simulink model "raspberry_pi_interface"  (R2023a)
settings: Solver=FixedStepDiscrete  StartTime=0.0  StopTime=inf  FixedStep=0.005  RelTol=1e-3  EnableMultiTasking=on
libraries: raspberrypiNetworklib x2, etargetslib x1
settings Model: SimulationMode=external  ExtModeTrigDuration=2  Creator=somml  LastModifiedBy=somml
settings SolverCC: AlgebraicLoopSolver=TrustRegion  PositivePriorityOrder=on
settings DataIOCC: ReturnWorkspaceOutputs=off
settings OptimizationCC: MaxStackSize=64
settings DebuggingCC: ParameterTunabilityLossMsg=error  UnconnectedInputMsg=warning  UnconnectedOutputMsg=warning  UnconnectedLineMsg=warning  ArithmeticOperatorsInVariantConditions=warning
settings HardwareCC: ProdBitPerPointer=32  ProdBitPerSizeT=32  ProdBitPerPtrDiffT=32  ProdLargestAtomicInteger=Long  ProdLargestAtomicFloat=Double  ProdWordSize=32  ProdHWDeviceType=ARM Compatible->ARM Cortex  UseEmbeddedCoderFeatures=off
settings ModelReferenceCC: EnableRefExpFcnMdlSchedulingChecks=on
settings SFSimCC: SimUseLocalCustomCode=off  CustomCodeUndefinedFunction=UseInterfaceOnly
settings RTWCC: Description=Embedded Coder  SystemTargetFile=ert.tlc  HardwareBoard=Raspberry Pi  TLCOptions="-aInlineSetEventsForThisBaseRateFcn=TLC_FALSE -aSuppressMultiTaskScheduler=TLC_FALSE  -aRateBasedStepFcn=0"  TemplateMakefile=ert_default_tmf  GenerateReport=on  RTWUseLocalCustomCode=off  Toolchain=GNU GCC Embedded Linux  BuildConfiguration=Faster Runs  LaunchReport=on  DLArmComputeVersion=19.05
settings CodeAppCC: ForceParamTrailComments=on  OperatorAnnotations=on  StateflowObjectComments=on  MATLABSourceComments=on
settings ERTTargetCC: TargetLangStandard=C99 (ISO)  ERTCustomFileBanners=off  SupportContinuousTime=on  SupportNonInlinedSFcns=on  RemoveResetFunc=off  SupportVariableSizeSignals=on  ModelStepFunctionPrototypeControlCompliant=off

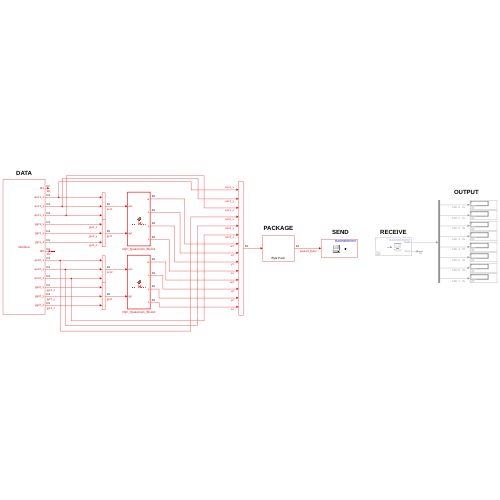
[thumbnail: Simulink's stored preview of the top-level diagram]
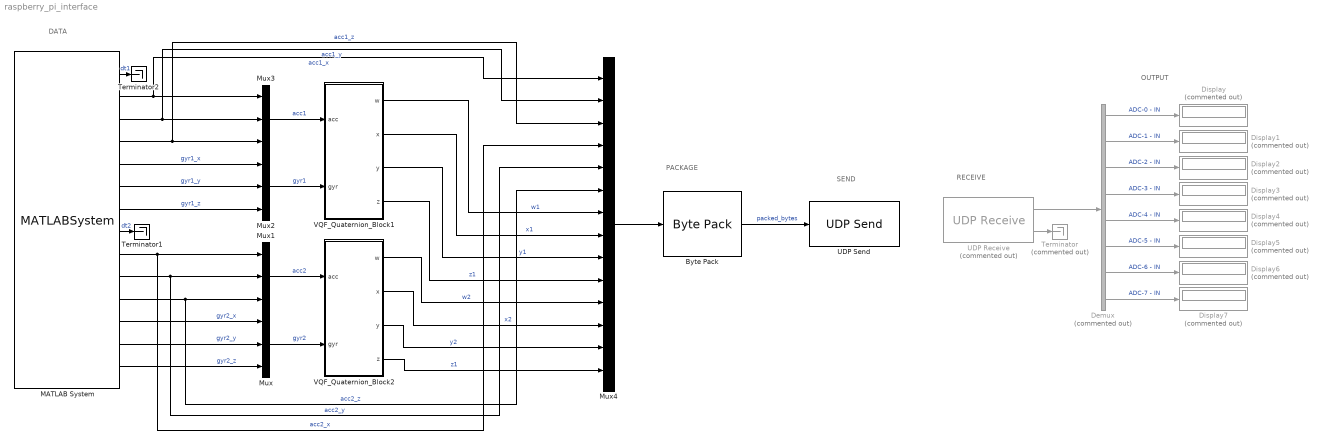
== system raspberry_pi_interface ==
  note: SEND
  note: RECEIVE
  note: DATA
  note: PACKAGE
  note: OUTPUT
  Byte Pack : etargetslib/Byte Pack  datatypes={'double'}  byteAlign=1
  Demux : Demux  Commented=on  Outputs=8
  Display{,1..7} (8 alike) : Display  Commented=on
  MATLAB System : MATLABSystem  System=interface  UpdateRateInHertz=200.0  SPIModuleBusSpeedInHz=500000  SimulateUsing=Code generation
      mask Type: interface
      mask Display:
      | disp('interface');
      | port_label('output',1,'dt1');
      | port_label('output',2,'acc1_x');
      | port_label('output',3,'acc1_y');
      | port_label('output',4,'acc1_z');
      | port_label('output',5,'gyr1_x');
      | port_label('output',6,'gyr1_y');
      | port_label('output',7,'gyr1_z');
      | port_label('output',8,'dt2');
      | port_label('output',9,'acc2_x');
      | port_label('output',10,'acc2_y');
      | port_label('output',11,'acc2_z');
      | port_label('output',12,'gyr2_x');
      | port_label('output',13,'gyr2_y');
      | port_label('output',14,'gyr2_z');
  Mux{,1..3} (4 alike) : Mux  Inputs=3
  Mux4 : Mux  Inputs=14
  Terminator : Terminator  Commented=on
  Terminator1 : Terminator
  Terminator2 : Terminator
  UDP Receive : raspberrypiNetworklib/UDP Receive  Commented=on  localURL='0.0.0.0'  localPort=8001  remoteURL='0.0.0.0'  remotePort=-1  recvBufferSize=8192  signalDatatype=double  dims=8  isVarSize=off  showBlockingTime=off  blockingTime=0  sampletime=0.005  blockPlatform=Raspberry Pi
  UDP Send : raspberrypiNetworklib/UDP Send  remoteURL='192.168.1.2'  remotePort=8000  localURL='0.0.0.0'  localPortSource=Automatically determine  localPort=-1  sampletime=-1  blockPlatform=Raspberry Pi  separateLengthPort=0
  VQF_Quaternion_Block1 : MATLAB Function  TreatAsAtomicUnit=on
  VQF_Quaternion_Block2 : MATLAB Function  TreatAsAtomicUnit=on
  wires:
  UDP Receive/2 -> Terminator/1
  UDP Receive/1 -> Demux/1
  Byte Pack/1 -> UDP Send/1  "packed_bytes"
  Demux/1 -> Display/1  "ADC-0 - IN"
  Demux/2 -> Display1/1  "ADC-1 - IN"
  Demux/3 -> Display2/1  "ADC-2 - IN"
  Demux/4 -> Display3/1  "ADC-3 - IN"
  Demux/5 -> Display4/1  "ADC-4 - IN"
  Demux/6 -> Display5/1  "ADC-5 - IN"
  Demux/7 -> Display6/1  "ADC-6 - IN"
  Demux/8 -> Display7/1  "ADC-7 - IN"
  MATLAB System/12 -> Mux/1  "gyr2_x"
  MATLAB System/13 -> Mux/2  "gyr2_y"
  MATLAB System/14 -> Mux/3  "gyr2_z"
  MATLAB System/10 -> Mux4/5, Mux1/2  "acc2_y"
  MATLAB System/9 -> Mux4/4, Mux1/1  "acc2_x"
  MATLAB System/11 -> Mux4/6, Mux1/3  "acc2_z"
  MATLAB System/2 -> Mux4/1, Mux3/1  "acc1_x"
  MATLAB System/3 -> Mux4/2, Mux3/2  "acc1_y"
  MATLAB System/4 -> Mux4/3, Mux3/3  "acc1_z"
  MATLAB System/5 -> Mux2/1  "gyr1_x"
  MATLAB System/6 -> Mux2/2  "gyr1_y"
  MATLAB System/7 -> Mux2/3  "gyr1_z"
  Mux3/1 -> VQF_Quaternion_Block1/1(acc)  "acc1"
  Mux2/1 -> VQF_Quaternion_Block1/2(gyr)  "gyr1"
  Mux1/1 -> VQF_Quaternion_Block2/1(acc)  "acc2"
  Mux/1 -> VQF_Quaternion_Block2/2(gyr)  "gyr2"
  MATLAB System/8 -> Terminator1/1  "dt2"
  MATLAB System/1 -> Terminator2/1  "dt1"
  VQF_Quaternion_Block1/1(w) -> Mux4/7  "w1"
  VQF_Quaternion_Block1/2(x) -> Mux4/8  "x1"
  VQF_Quaternion_Block1/3(y) -> Mux4/9  "y1"
  VQF_Quaternion_Block1/4(z) -> Mux4/10  "z1"
  VQF_Quaternion_Block2/1(w) -> Mux4/11  "w2"
  VQF_Quaternion_Block2/2(x) -> Mux4/12  "x2"
  VQF_Quaternion_Block2/3(y) -> Mux4/13  "y2"
  VQF_Quaternion_Block2/4(z) -> Mux4/14  "z1"
  Mux4/1 -> Byte Pack/1

== matlab function raspberry_pi_interface/VQF_Quaternion_Block2 ==
  data: acc input; gyr input; w output; x output; y output; z output
function [w, x, y, z] = vqf_block(acc, gyr)
    persistent vqf
    
    if isempty(vqf)
        vqf = VQF(0.005, struct('magDistRejectionEnabled', false));
    end

    vqf.update(gyr', acc');
    out = vqf.getQuat6D();
    w = out(1);
    x = out(2);
    y = out(3);
    z = out(4);
end

== matlab function raspberry_pi_interface/VQF_Quaternion_Block1 ==
  data: acc input; gyr input; w output; x output; y output; z output
function [w, x, y, z] = vqf_block(acc, gyr)
    persistent vqf
    
    if isempty(vqf)
        vqf = VQF(0.005, struct('magDistRejectionEnabled', false));
    end

    vqf.update(gyr', acc');
    out = vqf.getQuat6D();
    w = out(1);
    x = out(2);
    y = out(3);
    z = out(4);
end
